simulink library "G_IR_function"  (R2025b)
settings: Solver=VariableStepAuto  StartTime=0.0  StopTime=10.0  RelTol=1e-3
settings Model: Creator=cdt  LastModifiedBy=Chris

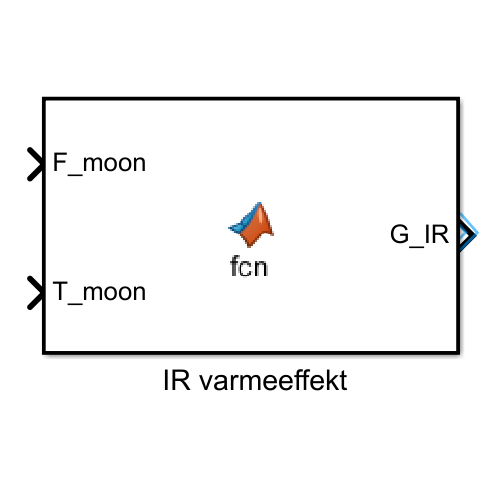
[thumbnail: Simulink's stored preview of the top-level diagram]
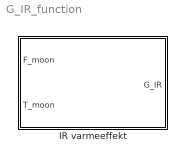
== system G_IR_function ==
  " IR varmeeffekt" : MATLAB Function  TreatAsAtomicUnit=on

== matlab function G_IR_function/ IR varmeeffekt ==
  data: G_IR output; F_moon input; T_moon input
function G_IR = fcn(F_moon, T_moon)
% G_IR: bestrålingseffekt af overflade (W/M^2)
% eps_surf: IR-emissivitet (absorptans) af roverens overflade
% A: areal af roverens overflade (m^2)
% F_moon: view factor til månen (0 til 1)
% T_moon: månens lokale overfladetemperatur (K)


sigma = 5.670e-8; % Stefan-Boltzmann konstant (W/(m^2*K^4))
epsilon_moon = 0.95; % månens emissivitet

% Beregn den absorberede infrarøde varmestråling fra måneoverfladen
G_IR = sigma * epsilon_moon * F_moon * (T_moon)^4;
